simulink model "sf_car"  (Simulink 6.0)
settings: Solver=ode5  SolverMode=SingleTasking  StartTime=0.0  StopTime=30  RelTol=1e-3  AbsTol=1e-6
PreLoadFcn:
  | load sf_cardat
values from neighbouring files (symbols this model uses):
  converter_data = [0 0.1 0.2 0.3 0.4 0.5 0.6 0.7 0.8 0.81 0.82 0.83 ... (63 elements, 21x3)]    [sf_cardat.mat]
  downtab = [0 0 0 0 0 0 5 5 5 5 30 30 ... (24 elements, 6x4)]    [sf_cardat.mat]
  emap = [-40 215 245 264 264 267 267 267 267 267 -44 117 ... (110 elements, 10x11)]    [sf_cardat.mat]
  Iei = 0.0219914882836    [sf_cardat.mat]
  uptab = [10 10 15 23 40 40 30 30 30 41 70 70 ... (24 elements, 6x4)]    [sf_cardat.mat]
undefined symbols (not defined in the file or in its folder): sigbuilder_block
settings Model: CovMetricSettings=dcmtr  Creator=The MathWorks Inc.  LastModifiedBy=batserve  ExtModeTrigMode=oneshot  ExtModeArmWhenConnect=off  ExtModeAutoUpdateStatusClock=off
settings DataIOCC: LimitDataPoints=off  SaveOutput=off  SaveTime=off  SignalLoggingName=sigsOut
settings OptimizationCC: BlockReduction=off  BooleanDataType=off
settings DebuggingCC: CheckExecutionContextPreStartOutputMsg=on  CheckExecutionContextRuntimeOutputMsg=on  SolverPrmCheckMsg=none  IntegerOverflowMsg=none
settings HardwareCC: TargetUnknown=on

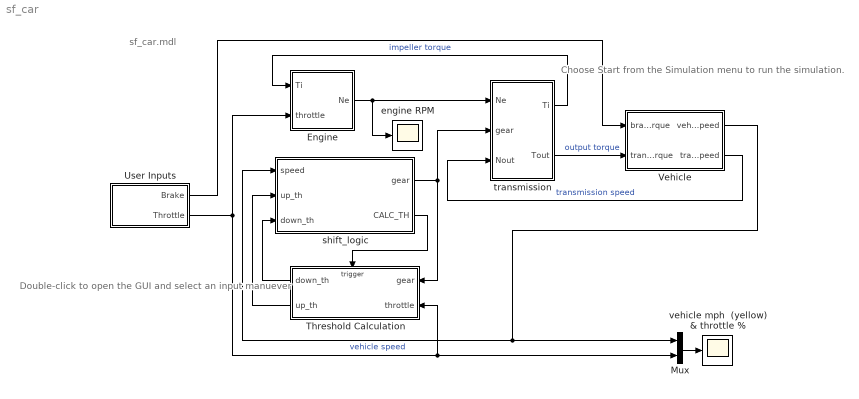
== system sf_car ==
  note: Choose Start from
      | the Simulation menu
      | to run the simulation.
  note: sf_car.mdl
  note: Double-click to
      | open the GUI
      | and select an
      | input manuever
  Engine : Subsystem  PropExecContextAcrossSSBoundary=on
  Mux : Mux  Inputs=2
  Threshold Calculation : Subsystem  Orientation=left  TreatAsAtomicUnit=on  PropExecContextAcrossSSBoundary=on
  User Inputs : Subsystem  Tag=STV Subsys  LoadFcn=sigbuilder_block('load');  StartFcn=sigbuilder_block('start');  StopFcn=sigbuilder_block('stop');  ClipboardFcn=sigbuilder_block('clipboard');  PropExecContextAcrossSSBoundary=on  mask(Sigbuilder block){}
      mask help: Sigbuilder GUI
      mask init:
      | tuvar = sigbuilder_block('maskInit');
      settings: CopyFcn=sigbuilder_block('copy');  DeleteFcn=sigbuilder_block('delete');  ModelCloseFcn=sigbuilder_block('modelClose');  PreSaveFcn=sigbuilder_block('preSave');  NameChangeFcn=sigbuilder_block('namechange');  OpenFcn=sigbuilder_block('open',[6 24.75 413.25 257.25 ]);  CloseFcn=sigbuilder_block('close');
      mask Display: plot(0,0,100,100,[10,10,40,40,10],[80,20,20,80,80],[40,10],[50,50], [40,27,10],[65,72,56],[40,25,25,10],[28,28,43,43]);
  Vehicle : Subsystem  PropExecContextAcrossSSBoundary=on  mask(vehicle model){@1=vehicledata(1), @2=vehicledata(2), @3=vehicledata(3), @4=vehicledata(4), @5=vehicledata(5), @6=vehicledata(6)/vehicledata(4)*vehicledata(1)}
      mask prompts: @1 "final drive ratio"; @2 "drag friction at wheels"; @3 "aerodynamic drag"; @4 "wheel radius"; @5 "vehicle inertia"; @6 "initial transmission output speed"
      mask help: vehicle dynamics: torque input from trans., outputs are input speed (transmission output) and vehicle speed
      mask init:
      | Rfd = @1; rload0 = @2; rload2 = @3; Rw = @4; Iv = @5; N20 = @6;
      mask Display: plot([cos(pi*[0:5:360]/180) + 6], [sin(pi*[0:5:360]/180) + 1.5],[cos(pi*[0:5:360]/180) + 1], [sin(pi*[0:5:360]/180) + 4], [10 7.5 6.75], [3.5 1 1.5], [10 9.75 7.5 6.25 3 1.5 4 5 7.5], [3.5 4.75 5.5 7 8 7 6 4 5.5], [6.5 4], [7 6], [5.25 2], [2 4], [7.5 1 0], [2.5 6 6.5], [7.5 7.25 9.75], [1 2.25 4.75], [2.75 2 0 0 0.25], [7.5 8 6.5 5.25 5], [1.5 0.5], [6.75 6.25])
  engine RPM : Scope
      settings: TickLabels=on  YMin=0  YMax=6000  DataFormat=Array
  shift_logic : Stateflow chart  PropExecContextAcrossSSBoundary=on
  transmission : Subsystem  PropExecContextAcrossSSBoundary=on
  vehicle mph  (yellow) & throttle % : Scope
      settings: TickLabels=on  YMin=0  YMax=140  DataFormat=Array
  wires:
  transmission/1(Ti) -> Engine/1(Ti)  "impeller torque"
  User Inputs/2(Throttle) -> Engine/2(throttle), Mux/2, Threshold Calculation/2(throttle)
  Engine/1(Ne) -> transmission/1(Ne), engine RPM/1
  transmission/2(Tout) -> Vehicle/2(transmission output torque)  "output torque"
  Vehicle/2(transmission output speed) -> transmission/3(Nout)  "transmission speed"
  Threshold Calculation/1(down_th) -> shift_logic/3(down_th)
  Threshold Calculation/2(up_th) -> shift_logic/2(up_th)
  shift_logic/1(gear) -> transmission/2(gear), Threshold Calculation/1(gear)
  shift_logic/2(CALC_TH) -> Threshold Calculation/Trigger
  Vehicle/1(vehicle speed) -> Mux/1, shift_logic/1(speed)  "vehicle speed"
  Mux/1 -> vehicle mph  (yellow) & throttle %/1
  User Inputs/1(Brake) -> Vehicle/1(brake torque)

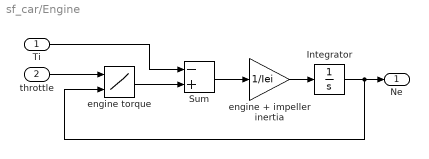
== system sf_car/Engine ==
  Ti : Inport  Port=1  LatchInput=off
  throttle : Inport  Port=2  LatchInput=off
  Integrator : Integrator  InitialCondition=1000  LimitOutput=on  UpperSaturationLimit=6000  LowerSaturationLimit=600  ZeroCross=off
  Sum : Sum  Inputs=-+  SaturateOnIntegerOverflow=on  InputSameDT=on
  engine torque : Lookup2D  DialogController=Simulink.DDGSource  RowIndex=thvec  ColumnIndex=nevec  OutputValues=emap  OutScaling=2^-10  InputSameDT=on
  engine + impeller inertia : Gain  Gain=1/Iei  SaturateOnIntegerOverflow=on
  Ne : Outport  InitialOutput=0
  wires:
  Ti/1 -> Sum/1
  throttle/1 -> engine torque/1
  Integrator/1 -> engine torque/2, Ne/1
  Sum/1 -> engine + impeller inertia/1
  engine + impeller inertia/1 -> Integrator/1
  engine torque/1 -> Sum/2

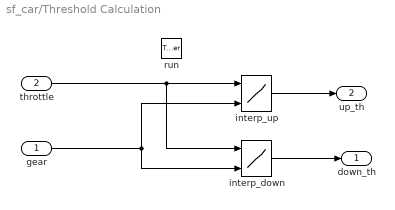
== system sf_car/Threshold Calculation ==
  gear : Inport  Port=1  LatchInput=off
  throttle : Inport  Port=2  LatchInput=off
  run : TriggerPort  TriggerType=function-call  ZeroCross=off
  interp_down : Lookup2D  DialogController=Simulink.DDGSource  RowIndex=downth  ColumnIndex=[1:4]  OutputValues=downtab  OutScaling=2^-10  InputSameDT=on
  interp_up : Lookup2D  DialogController=Simulink.DDGSource  RowIndex=upth  ColumnIndex=[1:4]  OutputValues=uptab  OutScaling=2^-10  InputSameDT=on
  down_th : Outport
  up_th : Outport  Port=2
  wires:
  interp_up/1 -> up_th/1
  interp_down/1 -> down_th/1
  throttle/1 -> interp_up/1, interp_down/1
  gear/1 -> interp_up/2, interp_down/2

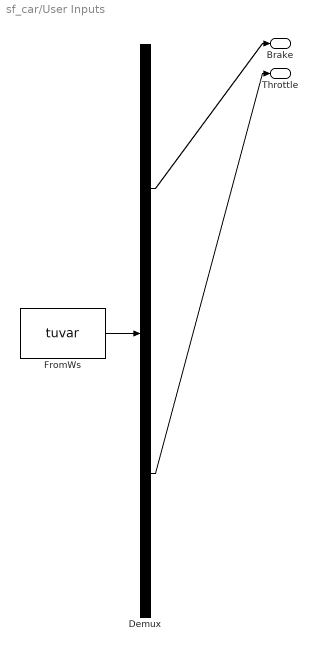
== system sf_car/User Inputs ==
  Demux : Demux  Tag=STV Demux  Outputs=2
  FromWs : FromWorkspace  Tag=STV FromWs  VariableName=tuvar  SampleTime=0  SigBuilderData=DataTag0  VnvData=DataTag1
      SigBuilderData=|
      | channels(1).label = 'Brake'
      | channels(1).allXData = {[0 50], [0 50], [0 10 10 50], [0 50]}
      | channels(1).allYData = {[0 0], [0 0], [0 0 325 325], [0 0]}
      | channels(2).label = 'Throttle'
      | channels(2).allXData = {[0 14.9 15 15 50], [0 50], [0 5.1 5.1 50], [0 4.8 4.8 50]}
      | channels(2).allYData = {[60 40 100 100 58.8235294118], [13.4 24], [50 50 1 1], [80 80 1 1]}
      | dataSet(1).timeRange = [0 50]
      | dataSet(1).name = 'Passing Maneuver'
      | dataSet(2).timeRange = [0 50]
      | dataSet(2).name = 'Gradual Acceleration'
      | dataSet(3).timeRange = [0 50]
      | dataSet(3).name = 'Hard braking'
      | dataSet(4).timeRange = [0 50]
      | dataSet(4).name = 'Coasting'
  Brake : Outport  Tag=STV Outport
  Throttle : Outport  Tag=STV Outport  Port=2
  wires:
  FromWs/1 -> Demux/1
  Demux/1 -> Brake/1
  Demux/2 -> Throttle/1

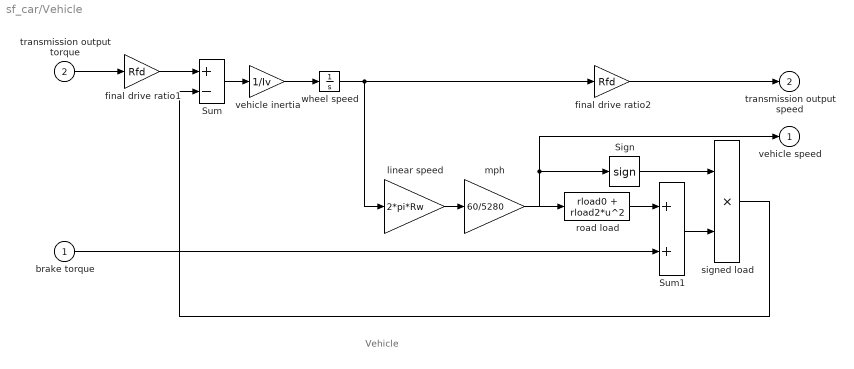
== system sf_car/Vehicle ==
  note: Vehicle
  brake torque : Inport  Port=1  LatchInput=off
  transmission output torque : Inport  Port=2  LatchInput=off
  Sign : Signum
  Sum : Sum  Inputs=+-  SaturateOnIntegerOverflow=on  InputSameDT=on
  Sum1 : Sum  SaturateOnIntegerOverflow=on  InputSameDT=on
  final drive ratio1 : Gain  Gain=Rfd  SaturateOnIntegerOverflow=on
  final drive ratio2 : Gain  Gain=Rfd  SaturateOnIntegerOverflow=on
  linear speed : Gain  Gain=2*pi*Rw  SaturateOnIntegerOverflow=on
  mph : Gain  Gain=60/5280  SaturateOnIntegerOverflow=on
  road load : Fcn  Expr=rload0 + rload2*u^2
  signed load : Product  SaturateOnIntegerOverflow=on  InputSameDT=on
  vehicle inertia : Gain  Gain=1/Iv  SaturateOnIntegerOverflow=on
  wheel speed : Integrator  InitialCondition=N20/Rfd  ZeroCross=off
  vehicle speed : Outport  InitialOutput=0
  transmission output speed : Outport  Port=2  InitialOutput=0
  wires:
  final drive ratio2/1 -> transmission output speed/1
  brake torque/1 -> Sum1/2
  Sum1/1 -> signed load/2
  road load/1 -> Sum1/1
  Sign/1 -> signed load/1
  signed load/1 -> Sum/2
  transmission output torque/1 -> final drive ratio1/1
  vehicle inertia/1 -> wheel speed/1
  Sum/1 -> vehicle inertia/1
  mph/1 -> vehicle speed/1, Sign/1, road load/1
  linear speed/1 -> mph/1
  wheel speed/1 -> linear speed/1, final drive ratio2/1
  final drive ratio1/1 -> Sum/1

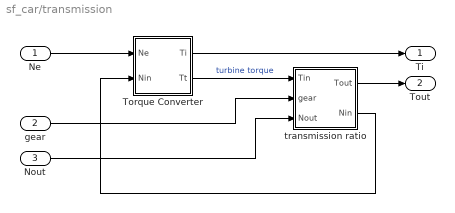
== system sf_car/transmission ==
  Ne : Inport  Port=1  LatchInput=off
  gear : Inport  Port=2  LatchInput=off
  Nout : Inport  Port=3  LatchInput=off
  Torque Converter : Subsystem  PropExecContextAcrossSSBoundary=on  mask(torque converter){speedratio=converter_data(:,1), Kfactor=converter_data(:,2), Torkratio=converter_data(:,3)}
      mask prompts: speedratio "speed ratio"; Kfactor "K factor"; Torkratio "torque ratio"
      mask help: torque converter
      mask Help: Torque converter input and output torques are computed as a function of the input and output speeds
      mask Display: plot([cos([90:10:450]*pi/180),.63*cos([90:10:450]*pi/180),.63*cos([90:10:240]*pi/180),cos([240:10:300]*pi/180),.63*cos([300]*pi/180)],[sin([90:10:450]*pi/180),.63*sin([90:10:450]*pi/180)+.1,.63*sin([90:10:240]*pi/180)+.1,sin([240:10:300]*pi/180),.63*sin([300]*pi/180)+.1])
  transmission ratio : Subsystem  PropExecContextAcrossSSBoundary=on
  Ti : Outport  InitialOutput=0
  Tout : Outport  Port=2  InitialOutput=0
  wires:
  transmission ratio/1(Tout) -> Tout/1
  Torque Converter/1(Ti) -> Ti/1
  Nout/1 -> transmission ratio/3(Nout)
  gear/1 -> transmission ratio/2(gear)
  Ne/1 -> Torque Converter/1(Ne)
  transmission ratio/2(Nin) -> Torque Converter/2(Nin)
  Torque Converter/2(Tt) -> transmission ratio/1(Tin)  "turbine torque"

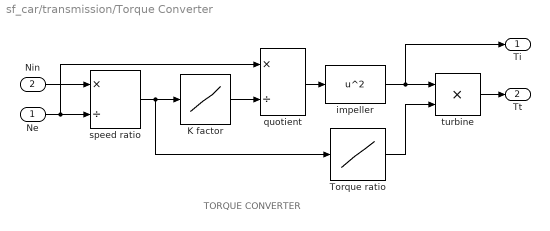
== system sf_car/transmission/Torque Converter ==
  note: TORQUE CONVERTER
  Ne : Inport  Port=1  LatchInput=off
  Nin : Inport  Port=2  LatchInput=off
  K factor : Lookup  DialogController=Simulink.DDGSource  InputValues=speedratio  OutputValues=Kfactor  SaturateOnIntegerOverflow=on
  Torque ratio : Lookup  DialogController=Simulink.DDGSource  InputValues=speedratio  OutputValues=Torkratio  SaturateOnIntegerOverflow=on
  impeller : Fcn  Expr=u^2
  quotient : Product  Inputs=*/  SaturateOnIntegerOverflow=on  InputSameDT=on
  speed ratio : Product  Inputs=*/  SaturateOnIntegerOverflow=on  InputSameDT=on
  turbine : Product  SaturateOnIntegerOverflow=on  InputSameDT=on
  Ti : Outport  InitialOutput=0
  Tt : Outport  Port=2  InitialOutput=0
  wires:
  Torque ratio/1 -> turbine/2
  quotient/1 -> impeller/1
  K factor/1 -> quotient/2
  speed ratio/1 -> Torque ratio/1, K factor/1
  impeller/1 -> turbine/1, Ti/1
  turbine/1 -> Tt/1
  Ne/1 -> speed ratio/2, quotient/1
  Nin/1 -> speed ratio/1

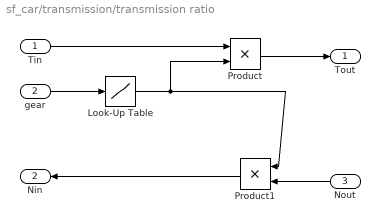
== system sf_car/transmission/transmission ratio ==
  Tin : Inport  Port=1  LatchInput=off
  gear : Inport  Port=2  LatchInput=off
  Nout : Inport  Orientation=left  Port=3  LatchInput=off
  Look-Up Table : Lookup  DialogController=Simulink.DDGSource  InputValues=[1 2 3 4]  OutputValues=[2.393 1.450 1.000 0.677]  SaturateOnIntegerOverflow=on
  Product : Product  SaturateOnIntegerOverflow=on  InputSameDT=on
  Product1 : Product  Orientation=left  SaturateOnIntegerOverflow=on  InputSameDT=on
  Tout : Outport  InitialOutput=0
  Nin : Outport  Orientation=left  Port=2  InitialOutput=0
  wires:
  Look-Up Table/1 -> Product1/1, Product/2
  Nout/1 -> Product1/2
  Product1/1 -> Nin/1
  Product/1 -> Tout/1
  Tin/1 -> Product/1
  gear/1 -> Look-Up Table/1

== stateflow chart shift_logic ==
  settings: updateMethod=DISCRETE  sampleTime=0.04
  state gear_state [parallel]
    state fourth
      entry: gear = 4;
    state second
      entry: gear = 2;
    state third
      entry: gear = 3;
    state first
      entry: gear = 1;
    third -> fourth : UP
    second -> third : UP
    first -> second : UP
    (default) -> first
    fourth -> third : DOWN
    third -> second : DOWN
    second -> first : DOWN
  state selection_state [parallel]
    during: CALC_TH;
    state downshifting
    state upshifting
    state steady_state
    (default) -> steady_state
    steady_state -> upshifting : [speed > up_th]
    steady_state -> downshifting : [speed < down_th]
    upshifting -> steady_state : [speed < up_th]
    downshifting -> steady_state : [speed > down_th]
    downshifting -> steady_state : after(TWAIT,tick)
        | [speed <= down_th]
        | {gear_state.DOWN}
    upshifting -> steady_state : after(TWAIT,tick)
        | [speed >= up_th]
        | {gear_state.UP}
  data: speed input double size=1; gear output uint8 size=1 [1..4]; TWAIT parameter uint8 size=1; up_th input double size=1; down_th input double size=1
  data speed settings: units=double
  data gear settings: units=int
  events: DOWN local EITHER_EDGE_EVENT; UP local EITHER_EDGE_EVENT; CALC_TH output FUNCTION_CALL_EVENT
